simulink library "SEMACE1_INSTRUMENTATION"  (R2021b)
settings: Solver=VariableStepAuto  StartTime=0.0  StopTime=10.0  RelTol=1e-3
settings Model: Creator=ACH  LastModifiedBy=ACH

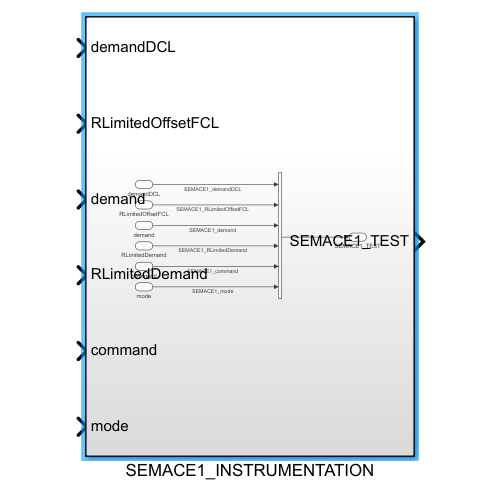
[thumbnail: Simulink's stored preview of the top-level diagram]
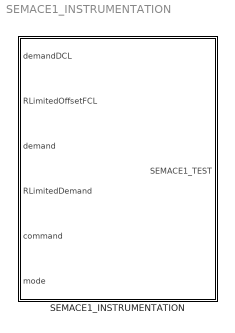
== system SEMACE1_INSTRUMENTATION ==
  SEMACE1_INSTRUMENTATION : Subsystem

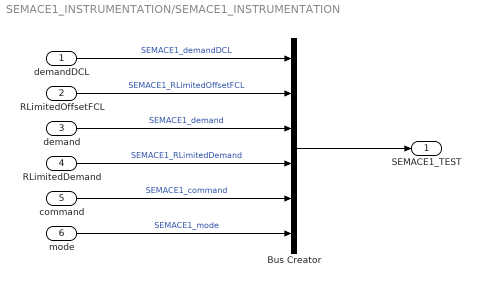
== system SEMACE1_INSTRUMENTATION/SEMACE1_INSTRUMENTATION ==
  demandDCL : Inport
  RLimitedOffsetFCL : Inport  Port=2
  demand : Inport  Port=3
  RLimitedDemand : Inport  Port=4
  command : Inport  Port=5
  mode : Inport  Port=6
  Bus Creator : BusCreator  Inputs=6  OutDataTypeStr=Bus: SEMACE1_TEST
  SEMACE1_TEST : Outport  OutDataTypeStr=Bus: SEMACE1_TEST
  wires:
  mode/1 -> Bus Creator/6  "SEMACE1_mode"
  demand/1 -> Bus Creator/3  "SEMACE1_demand"
  Bus Creator/1 -> SEMACE1_TEST/1
  command/1 -> Bus Creator/5  "SEMACE1_command"
  demandDCL/1 -> Bus Creator/1  "SEMACE1_demandDCL"
  RLimitedOffsetFCL/1 -> Bus Creator/2  "SEMACE1_RLimitedOffsetFCL"
  RLimitedDemand/1 -> Bus Creator/4  "SEMACE1_RLimitedDemand"
